simulink model "SVPWM_simulink"  (R2018a)
settings: Solver=VariableStepAuto  StartTime=0.0  StopTime=.06  FixedStep=2e-6  MaxStep=2e-6  RelTol=1e-3
libraries: powerlib x17, powerlib_meascontrol x1, peTransforms x1, simulink_extras x1
settings Model: Creator=ShahRukh  LastModifiedBy=ShahRukh

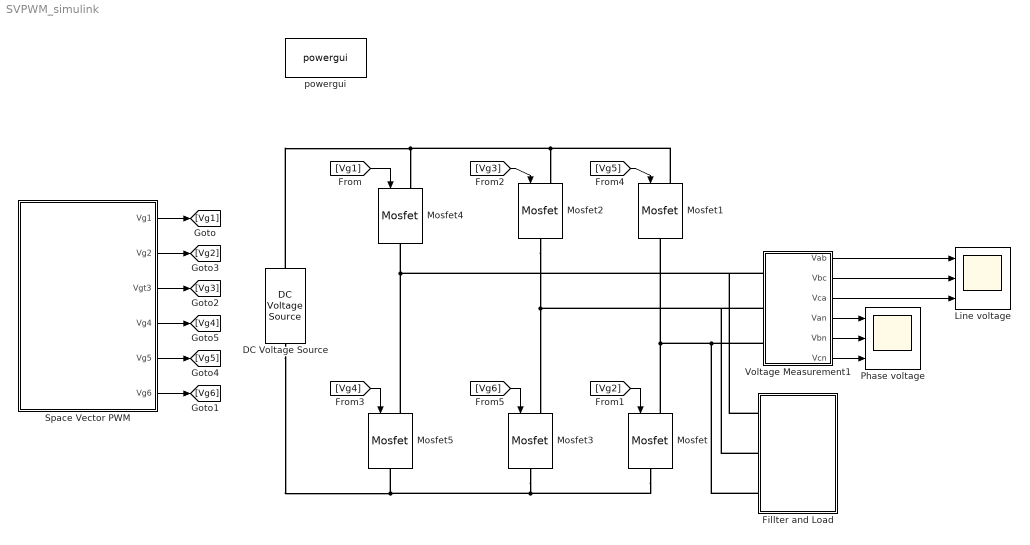
== system SVPWM_simulink ==
  DC Voltage Source : powerlib/Electrical Sources/DC Voltage Source  Amplitude=780  Measurements=None
  Fillter and Load : Subsystem
  Line voltage : Scope  NumInputPorts=3
  Mosfet{,1..5} (6 alike) : powerlib/Power Electronics/Mosfet  Ron=0.1  Lon=0  Rd=0.01  Vfd=0  IC=0  Rs=1e5  Cs=inf  Measurements=off
  Phase voltage : Scope  NumInputPorts=3
  Space Vector PWM : Subsystem
  Voltage Measurement1 : Subsystem
  powergui : powerlib/powergui  Priority=1  SimulationMode=Discrete  SampleTime=2e-6  frequency=60  Iterations=50  frequencyindice=0  Pbase=100e6  ErrMax=1e-4  UnitsV=kV  UnitsW=MW  buscounter=0  FunctionMessages=off  echomessages=off  EnableUseOfTLC=off  CurrentSourceSwitches=off  DisableSnubberDevices=off  DisableRonSwitches=off  DisableVfSwitches=off  DisplayEquations=off  SolverType=Tustin/Backward Euler (TBE)  Interpol=off  ExternalGateDelay=off  methode=off  Ts=100  x0status=blocks  SPID=off  SwTol=0  HookPort=off  RestoreLinks=warning  ResistiveCurrentMeasurement=off  Frange=[0:2:500]  Ylog=off  Xlog=on  ShowGrid=off  save=off  variable=ZData  structure=ScopeData3  ZoomFFT=off  StartTime=0.04  cycles=1  DisplayStyle=1  fundamental=50  FreqAxis=off  MaxFrequency=2000  frequencyindicesteady=1  RmsSteady=1  display=off
  wires:
  Space Vector PWM/6(Vg6) -> [Vg6]
  Space Vector PWM/4(Vg4) -> [Vg4]
  Space Vector PWM/3(Vgt3) -> [Vg3]
  [Vg1] -> Mosfet4/1
  [Vg2] -> Mosfet/1
  Space Vector PWM/1(Vg1) -> [Vg1]
  [Vg6] -> Mosfet3/1
  [Vg5] -> Mosfet1/1
  [Vg3] -> Mosfet2/1
  [Vg4] -> Mosfet5/1
  Space Vector PWM/5(Vg5) -> [Vg5]
  Space Vector PWM/2(Vg2) -> [Vg2]
  Voltage Measurement1/3(Vca) -> Line voltage/3
  Voltage Measurement1/4(Van) -> Phase voltage/1
  Voltage Measurement1/5(Vbn) -> Phase voltage/2
  Voltage Measurement1/2(Vbc) -> Line voltage/2
  Voltage Measurement1/1(Vab) -> Line voltage/1
  Voltage Measurement1/6(Vcn) -> Phase voltage/3
  connections:
  Mosfet/RConn1 -- Mosfet3/RConn1 -- DC Voltage Source/LConn1 -- Mosfet5/RConn1
  Mosfet1/LConn1 -- Mosfet2/LConn1 -- DC Voltage Source/RConn1 -- Mosfet4/LConn1
  Mosfet5/LConn1 -- Fillter and Load/LConn1 -- Voltage Measurement1/LConn1 -- Mosfet4/RConn1
  Mosfet2/RConn1 -- Fillter and Load/LConn2 -- Voltage Measurement1/LConn2 -- Mosfet3/LConn1
  Voltage Measurement1/LConn3 -- Fillter and Load/LConn3 -- Mosfet/LConn1 -- Mosfet1/RConn1

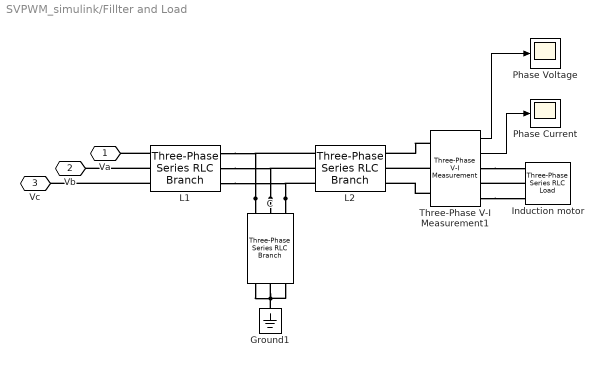
== system SVPWM_simulink/Fillter and Load ==
  C : powerlib/Elements/Three-Phase Series RLC Branch  LConnTagsString=A|B|C  RConnTagsString=A|B|C  BranchType=C  Resistance=1  Inductance=1e-3  Capacitance=1e-3  Measurements=None
  Ground1 : powerlib/Elements/Ground  LConnTagsString=a
  Induction motor : powerlib/Elements/Three-Phase Series RLC Load  LConnTagsString=A|B|C  Configuration=Y (grounded)  NominalVoltage=150  Vabc=[1e3 1e3 1e3]  Vabcp=[1e3 1e3 1e3]  NominalFrequency=50  UnbalancedPower=off  ActivePower=500  InductivePower=245  CapacitivePower=0  Pabc=[10e3 9e3 11e3]  QLabc=[100 90 110]  QCabc=[100 90 110]  Pabcp=[10e3 9e3 11e3]  QLabcp=[100 90 110]  QCabcp=[100 90 110]  Measurements=None  LoadType=constant Z
  L1 : powerlib/Elements/Three-Phase Series RLC Branch  LConnTagsString=A|B|C  RConnTagsString=A|B|C  BranchType=L  Resistance=1  Inductance=100e-6  Capacitance=1e-6  Measurements=None
  L2 : powerlib/Elements/Three-Phase Series RLC Branch  LConnTagsString=A|B|C  RConnTagsString=A|B|C  BranchType=L  Resistance=1  Inductance=100e-6  Capacitance=1e-6  Measurements=None
  Phase Current : Scope
  Phase Voltage : Scope
  Three-Phase V-I Measurement1 : powerlib/Measurements/Three-Phase V-I Measurement  VoltageMeasurement=phase-to-ground  SetLabelV=off  LabelV=Vabc  Vpu=off  VpuLL=off  CurrentMeasurement=yes  SetLabelI=off  LabelI=Iabc  Ipu=off  Pbase=100e6  Vbase=500e3  OutputType=Complex  PhasorSimulation=off  PSBequivalent=0
  Va : PMIOPort  Side=Left
  Vb : PMIOPort  Port=2  Side=Left
  Vc : PMIOPort  Port=3  Side=Left
  wires:
  Three-Phase V-I Measurement1/1 -> Phase Voltage/1
  Three-Phase V-I Measurement1/2 -> Phase Current/1
  connections:
  C/LConn2 -- L1/RConn2 -- L2/LConn2
  Three-Phase V-I Measurement1/LConn2 -- L2/RConn2
  C/LConn3 -- L1/RConn3 -- L2/LConn3
  C/LConn1 -- L1/RConn1 -- L2/LConn1
  Three-Phase V-I Measurement1/LConn3 -- L2/RConn3
  Three-Phase V-I Measurement1/LConn1 -- L2/RConn1
  C/RConn2 -- C/RConn1 -- C/RConn3 -- Ground1/LConn1
  Induction motor/LConn2 -- Three-Phase V-I Measurement1/RConn2
  Three-Phase V-I Measurement1/RConn1 -- Induction motor/LConn1
  Three-Phase V-I Measurement1/RConn3 -- Induction motor/LConn3
  L1/LConn3 -- Vc/RConn1
  L1/LConn2 -- Vb/RConn1
  L1/LConn1 -- Va/RConn1

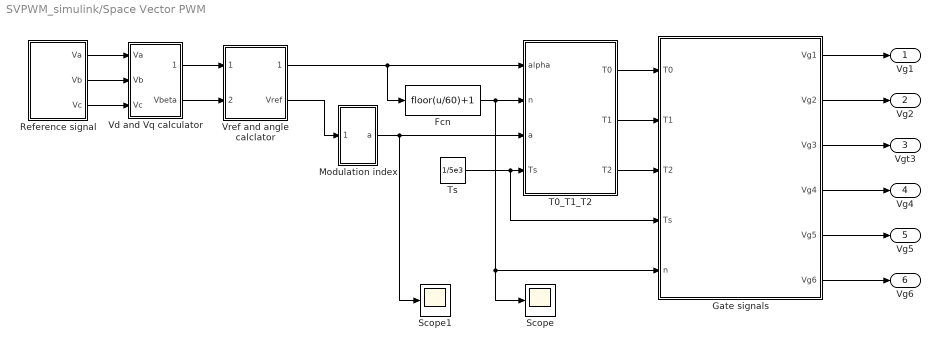
== system SVPWM_simulink/Space Vector PWM ==
  Fcn : Fcn  Expr=floor(u/60)+1
  Gate signals : Subsystem
  Modulation index : Subsystem
  Reference signal : Subsystem
  Scope : Scope
  Scope1 : Scope
  T0_T1_T2 : Subsystem
  Ts : Constant  Value=1/5e3
  Vd and Vq calculator : Subsystem
  Vref and angle calclator : Subsystem
  Vg1 : Outport
  Vg2 : Outport  Port=2
  Vgt3 : Outport  Port=3
  Vg4 : Outport  Port=4
  Vg5 : Outport  Port=5
  Vg6 : Outport  Port=6
  wires:
  Reference signal/2(Vb) -> Vd and Vq calculator/2(Vb)
  Fcn/1 -> T0_T1_T2/2(n), Scope/1, Gate signals/5(n)
  T0_T1_T2/3(T2) -> Gate signals/3(T2)
  Reference signal/3(Vc) -> Vd and Vq calculator/3(Vc)
  Gate signals/5(Vg5) -> Vg5/1
  Gate signals/6(Vg6) -> Vg6/1
  Gate signals/4(Vg4) -> Vg4/1
  Gate signals/3(Vg3) -> Vgt3/1
  Gate signals/1(Vg1) -> Vg1/1
  Reference signal/1(Va) -> Vd and Vq calculator/1(Va)
  Ts/1 -> Gate signals/4(Ts), T0_T1_T2/4(Ts)
  Gate signals/2(Vg2) -> Vg2/1
  T0_T1_T2/1(T0) -> Gate signals/1(T0)
  T0_T1_T2/2(T1) -> Gate signals/2(T1)
  Vd and Vq calculator/2(Vbeta) -> Vref and angle calclator/2(Vbeta)
  Vd and Vq calculator/1(Valpha) -> Vref and angle calclator/1(Valpha)
  Vref and angle calclator/2(Vref) -> Modulation index/1(Vref)
  Vref and angle calclator/1(alpha) -> Fcn/1, T0_T1_T2/1(alpha)
  Modulation index/1(a) -> Scope1/1, T0_T1_T2/3(a)

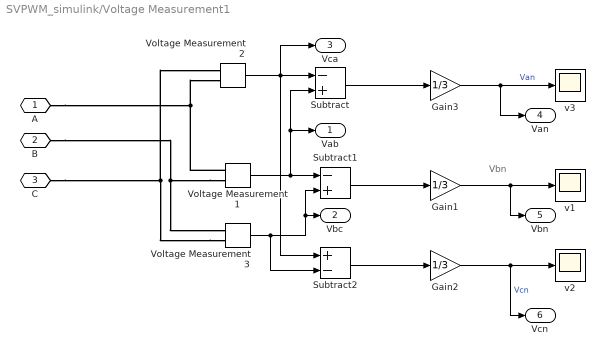
== system SVPWM_simulink/Voltage Measurement1 ==
  note: Vbn
  Gain1 : Gain  Gain=1/3
  Gain2 : Gain  Gain=1/3
  Gain3 : Gain  Gain=1/3
  Subtract : Sum  Inputs=-+
  Subtract1 : Sum  Inputs=-+
  Subtract2 : Sum  Inputs=+-
  Voltage Measurement1 : powerlib/Measurements/Voltage Measurement  PhasorSimulation=off  OutputType=Complex  PSBequivalent=0
  Voltage Measurement2 : powerlib/Measurements/Voltage Measurement  PhasorSimulation=off  OutputType=Complex  PSBequivalent=0
  Voltage Measurement3 : powerlib/Measurements/Voltage Measurement  PhasorSimulation=off  OutputType=Complex  PSBequivalent=0
  v1 : Scope
  v2 : Scope
  v3 : Scope
  A : PMIOPort  Side=Left
  B : PMIOPort  Port=2  Side=Left
  C : PMIOPort  Port=3  Side=Left
  Vab : Outport
  Vbc : Outport  Port=2
  Vca : Outport  Port=3
  Van : Outport  Port=4
  Vbn : Outport  Port=5
  Vcn : Outport  Port=6
  wires:
  Gain2/1 -> v2/1, Vcn/1  "Vcn"
  Subtract2/1 -> Gain2/1
  Gain1/1 -> v1/1, Vbn/1
  Subtract1/1 -> Gain1/1
  Voltage Measurement3/1 -> Subtract1/2, Vbc/1, Subtract2/2
  Gain3/1 -> v3/1, Van/1  "Van"
  Subtract/1 -> Gain3/1
  Voltage Measurement1/1 -> Vab/1, Subtract/2, Subtract1/1
  Voltage Measurement2/1 -> Vca/1, Subtract2/1, Subtract/1
  connections:
  Voltage Measurement1/LConn1 -- A/RConn1 -- Voltage Measurement2/LConn2
  Voltage Measurement1/LConn2 -- B/RConn1 -- Voltage Measurement3/LConn1
  Voltage Measurement3/LConn2 -- Voltage Measurement2/LConn1 -- C/RConn1

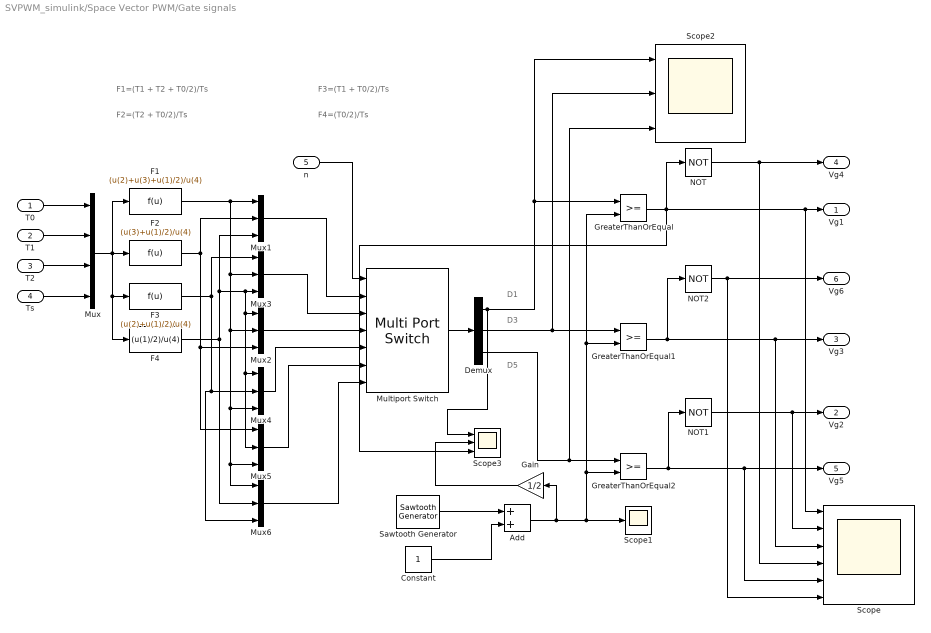
== system SVPWM_simulink/Space Vector PWM/Gate signals ==
  note: D1
  note: F1=(T1 + T2 + T0/2)/Ts
  note: F2=(T2 + T0/2)/Ts
  note: F3=(T1 + T0/2)/Ts
  note: F4=(T0/2)/Ts
  note: D3
  note: D5
  T0 : Inport
  T1 : Inport  Port=2
  T2 : Inport  Port=3
  Ts : Inport  Port=4
  n : Inport  Port=5
  Add : Sum
  Constant : Constant
  Demux : Demux  Outputs=3
  F1 : Fcn  Expr=(u(2)+u(3)+u(1)/2)/u(4)
  F2 : Fcn  Expr=(u(3)+u(1)/2)/u(4)
  F3 : Fcn  Expr=(u(2)+u(1)/2)/u(4)
  F4 : Fcn  Expr=(u(1)/2)/u(4)
  Gain : Gain  Gain=1/2
  GreaterThanOrEqual : RelationalOperator  OutDataTypeStr=boolean  RndMeth=Simplest
  GreaterThanOrEqual1 : RelationalOperator  OutDataTypeStr=boolean  RndMeth=Simplest
  GreaterThanOrEqual2 : RelationalOperator  OutDataTypeStr=boolean  RndMeth=Simplest
  Multiport Switch : MultiPortSwitch  Inputs=6  DiagnosticForDefault=None
  Mux : Mux
  Mux{1..6} (6 alike) : Mux  Inputs=3
  NOT : Logic  Operator=NOT  IconShape=distinctive  AllPortsSameDT=off  OutDataTypeStr=boolean
  NOT1 : Logic  Operator=NOT  IconShape=distinctive  AllPortsSameDT=off  OutDataTypeStr=boolean
  NOT2 : Logic  Operator=NOT  IconShape=distinctive  AllPortsSameDT=off  OutDataTypeStr=boolean
  Sawtooth Generator : powerlib_meascontrol/Pulse & Signal Generators/Sawtooth Generator  Freq=5e3  Phase=0  Ts=0
      settings: SourceProductName=Simscape Power Systems
  Scope : Scope  NumInputPorts=6
  Scope1 : Scope
  Scope2 : Scope  NumInputPorts=3
  Scope3 : Scope  NumInputPorts=3
  Vg1 : Outport
  Vg2 : Outport  Port=2
  Vg3 : Outport  Port=3
  Vg4 : Outport  Port=4
  Vg5 : Outport  Port=5
  Vg6 : Outport  Port=6
  wires:
  Demux/2 -> GreaterThanOrEqual1/1, Scope2/2
  Sawtooth Generator/1 -> Add/1
  GreaterThanOrEqual/1 -> Scope3/3, Scope/1, Vg1/1, NOT/1
  GreaterThanOrEqual1/1 -> NOT2/1, Scope/3, Vg3/1
  GreaterThanOrEqual2/1 -> NOT1/1, Scope/5, Vg5/1
  NOT/1 -> Scope/4, Vg4/1
  NOT1/1 -> Scope/2, Vg2/1
  NOT2/1 -> Scope/6, Vg6/1
  n/1 -> Multiport Switch/1
  T0/1 -> Mux/1
  T1/1 -> Mux/2
  T2/1 -> Mux/3
  Ts/1 -> Mux/4
  Mux/1 -> F1/1, F2/1, F4/1, F3/1
  Demux/3 -> GreaterThanOrEqual2/1, Scope2/3
  Add/1 -> Gain/1, Scope1/1, GreaterThanOrEqual2/2, GreaterThanOrEqual1/2, GreaterThanOrEqual/2
  Constant/1 -> Add/2
  Multiport Switch/1 -> Demux/1
  Demux/1 -> Scope3/1, GreaterThanOrEqual/1, Scope2/1
  Mux6/1 -> Multiport Switch/7
  Mux5/1 -> Multiport Switch/6
  Mux4/1 -> Multiport Switch/5
  Mux2/1 -> Multiport Switch/4
  Mux3/1 -> Multiport Switch/3
  Mux1/1 -> Multiport Switch/2
  F1/1 -> Mux6/1, Mux5/3, Mux4/3, Mux2/2, Mux3/2, Mux1/1
  F2/1 -> Mux1/2, Mux5/1, Mux2/3
  F4/1 -> Mux6/2, Mux5/2, Mux4/1, Mux2/1, Mux3/3, Mux1/3
  F3/1 -> Mux6/3, Mux4/2, Mux3/1
  Gain/1 -> Scope3/2

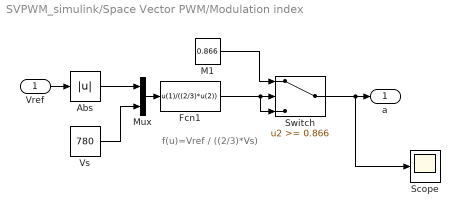
== system SVPWM_simulink/Space Vector PWM/Modulation index ==
  note: f(u)=Vref / ((2/3)*Vs)
  Vref : Inport
  Abs : Abs
  Fcn1 : Fcn  Expr=u(1)/((2/3)*u(2))
  M1 : Constant  Value=0.866
  Mux : Mux  Inputs=2
  Scope : Scope
  Switch : Switch  Threshold=0.866
  Vs : Constant  Value=780
  a : Outport
  wires:
  Fcn1/1 -> Switch/3, Switch/2
  Vs/1 -> Mux/2
  M1/1 -> Switch/1
  Vref/1 -> Abs/1
  Mux/1 -> Fcn1/1
  Switch/1 -> Scope/1, a/1
  Abs/1 -> Mux/1

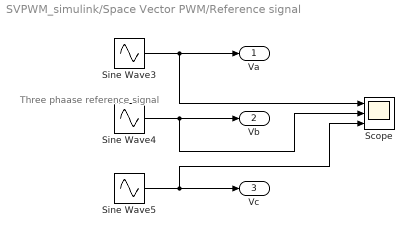
== system SVPWM_simulink/Space Vector PWM/Reference signal ==
  note: Three phaase
      | reference signal
  Scope : Scope  NumInputPorts=3
  Sine Wave3 : Sin  Amplitude=440  Frequency=2*pi*50  SampleTime=0
  Sine Wave4 : Sin  Amplitude=440  Frequency=2*pi*50  Phase=-2*pi/3  SampleTime=0
  Sine Wave5 : Sin  Amplitude=440  Frequency=2*pi*50  Phase=2*pi/3  SampleTime=0
  Va : Outport
  Vb : Outport  Port=2
  Vc : Outport  Port=3
  wires:
  Sine Wave4/1 -> Scope/2, Vb/1
  Sine Wave5/1 -> Scope/3, Vc/1
  Sine Wave3/1 -> Scope/1, Va/1

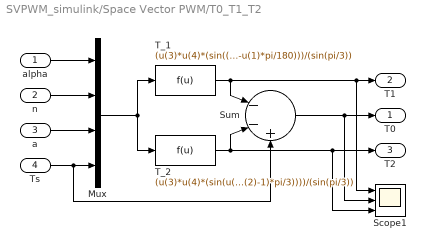
== system SVPWM_simulink/Space Vector PWM/T0_T1_T2 ==
  alpha : Inport
  n : Inport  Port=2
  a : Inport  Port=3
  Ts : Inport  Port=4
  Mux : Mux
  Scope1 : Scope  NumInputPorts=3
  Sum : Sum  Inputs=|--+
  T_1 : Fcn  Expr=(u(3)*u(4)*(sin((u(2)*pi/3)-u(1)*pi/180)))/(sin(pi/3))
  T_2 : Fcn  Expr=(u(3)*u(4)*(sin(u(1)*pi/180-((u(2)-1)*pi/3))))/(sin(pi/3))
  T0 : Outport
  T1 : Outport  Port=2
  T2 : Outport  Port=3
  wires:
  Mux/1 -> T_2/1, T_1/1
  n/1 -> Mux/2
  a/1 -> Mux/3
  Ts/1 -> Sum/3, Mux/4
  T_2/1 -> Sum/2, Scope1/3, T2/1
  T_1/1 -> Scope1/1, T1/1, Sum/1
  Sum/1 -> Scope1/2, T0/1
  alpha/1 -> Mux/1

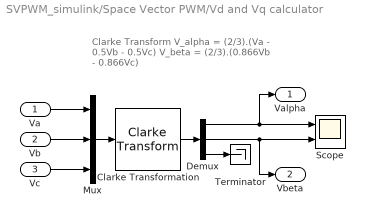
== system SVPWM_simulink/Space Vector PWM/Vd and Vq calculator ==
  note: Clarke Transform
      | V_alpha = (2/3).(Va - 0.5Vb - 0.5Vc)
      | V_beta = (2/3).(0.866Vb - 0.866Vc)
  Va : Inport
  Vb : Inport  Port=2
  Vc : Inport  Port=3
  Clarke Transformation : peTransforms/Clarke Transform  PowerInvariant=off
  Demux : Demux  Outputs=3
  Mux : Mux  Inputs=3
  Scope : Scope  NumInputPorts=2
  Terminator : Terminator
  Valpha : Outport
  Vbeta : Outport  Port=2
  wires:
  Va/1 -> Mux/1
  Vb/1 -> Mux/2
  Vc/1 -> Mux/3
  Mux/1 -> Clarke Transformation/1
  Clarke Transformation/1 -> Demux/1
  Demux/1 -> Scope/1, Valpha/1
  Demux/2 -> Scope/2, Vbeta/1
  Demux/3 -> Terminator/1

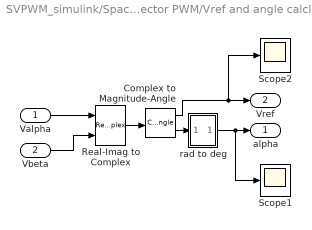
== system SVPWM_simulink/Space Vector PWM/Vref and angle calclator ==
  Valpha : Inport
  Vbeta : Inport  Port=2
  Complex to Magnitude-Angle : ComplexToMagnitudeAngle
  Real-Imag to Complex : RealImagToComplex
  Scope1 : Scope
  Scope2 : Scope
  rad to deg : Subsystem
  alpha : Outport
  Vref : Outport  Port=2
  wires:
  Valpha/1 -> Real-Imag to Complex/1
  Real-Imag to Complex/1 -> Complex to Magnitude-Angle/1
  Vbeta/1 -> Real-Imag to Complex/2
  rad to deg/1(2D) -> alpha/1, Scope1/1
  Complex to Magnitude-Angle/2 -> rad to deg/1(R)
  Complex to Magnitude-Angle/1 -> Scope2/1, Vref/1

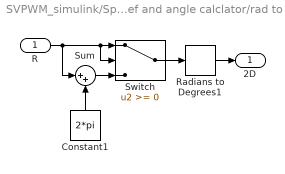
== system SVPWM_simulink/Space Vector PWM/Vref and angle calclator/rad to deg ==
  R : Inport
  Constant1 : Constant  Value=2*pi
  Radians to Degrees1 : simulink_extras/Transformations/Radians to Degrees
  Sum : Sum  Inputs=|++
  Switch : Switch
  2D : Outport
  wires:
  R/1 -> Switch/2, Switch/1, Sum/1
  Radians to Degrees1/1 -> 2D/1
  Switch/1 -> Radians to Degrees1/1
  Sum/1 -> Switch/3
  Constant1/1 -> Sum/2
